simulink model "biomass"  (R2017a)
settings: Solver=VariableStepAuto  StartTime=0.0  StopTime=300  RelTol=1e-3
undefined symbols (not defined in the file): ba, bh, fp
settings Model: Creator=pum  LastModifiedBy=pum

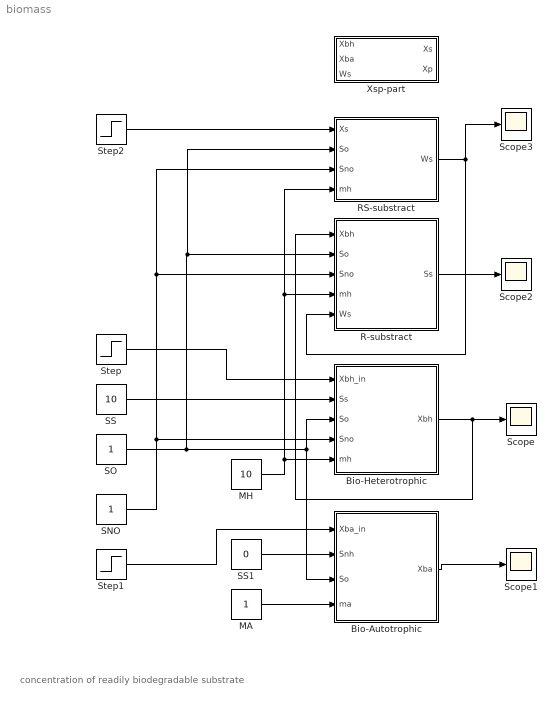
== system biomass ==
  note: concentration of readily biodegradable substrate
  Bio-Autotrophic : Subsystem  mask{Xba0=0, ba=1, Knh=3, Koa=5}
      mask prompts: Xba0 "Initialvalue"; ba "Ba cofficient"
  Bio-Heterotrophic : Subsystem  mask{Xbh0=0, bh=1, ng=1, Ks=0.1, Koh=0.1, Kno=0.3}
      mask prompts: Xbh0 "Initialvalue"; bh "Bh cofficient"; ng "Ng coefficient"
  MA : Constant
  MH : Constant  Value=10
  R-substract : Subsystem  mask{Y_h=50, ng=1, Ks=0.1, Koh=0.1, Kno=0.3}
  RS-substract : Subsystem  mask{kh=1, nh=1, Ks=0.1, Koh=0.1, Kno=0.3}
      mask prompts: nh "Ng"
  SNO : Constant
  SO : Constant
  SS : Constant  Value=10
  SS1 : Constant  Value=0
  Scope{,1..3} (4 alike) : Scope
  Step : Step  SampleTime=0
  Step1 : Step  SampleTime=0
  Step2 : Step  SampleTime=0
  Xsp-part : Subsystem
  wires:
  MH/1 -> RS-substract/4(mh), R-substract/4(mh), Bio-Heterotrophic/5(mh)
  SO/1 -> RS-substract/2(So), R-substract/2(So), Bio-Heterotrophic/3(So), Bio-Autotrophic/3(So)
  SNO/1 -> RS-substract/3(Sno), R-substract/3(Sno), Bio-Heterotrophic/4(Sno)
  Step/1 -> Bio-Heterotrophic/1(Xbh_in)
  MA/1 -> Bio-Autotrophic/4(ma)
  Step1/1 -> Bio-Autotrophic/1(Xba_in)
  Bio-Autotrophic/1(Xba) -> Scope1/1
  SS/1 -> Bio-Heterotrophic/2(Ss)
  SS1/1 -> Bio-Autotrophic/2(Snh)
  R-substract/1(Ss) -> Scope2/1
  Bio-Heterotrophic/1(Xbh) -> R-substract/1(Xbh), Scope/1
  RS-substract/1(Ws) -> Scope3/1, R-substract/5(Ws)
  Step2/1 -> RS-substract/1(Xs)

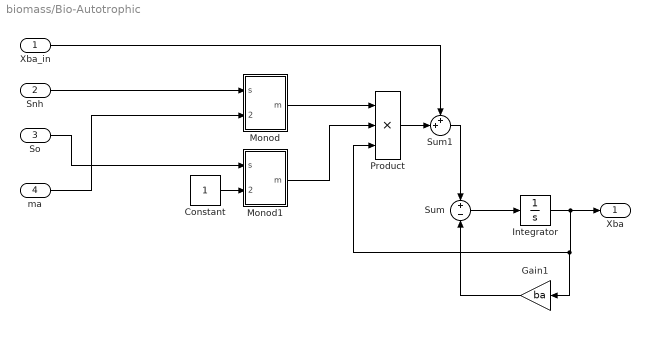
== system biomass/Bio-Autotrophic ==
  Xba_in : Inport
  Snh : Inport  Port=2
  So : Inport  Port=3
  ma : Inport  Port=4
  Constant : Constant
  Gain1 : Gain  Gain=ba
  Integrator : Integrator  InitialCondition=Xba0
  Monod : Subsystem  mask{K=Knh}
      mask prompts: K "Half-speed coeffcient"
  Monod1 : Subsystem  mask{K=Koa}
      mask prompts: K "Half-speed coeffcient"
  Product : Product  Inputs=3
  Sum : Sum  Inputs=+-
  Sum1 : Sum  Inputs=++|
  Xba : Outport
  wires:
  Integrator/1 -> Gain1/1, Product/3, Xba/1
  Snh/1 -> Monod/1(s)
  Monod1/1(m) -> Product/2
  Sum/1 -> Integrator/1
  Product/1 -> Sum1/2
  ma/1 -> Monod/2(m_max)
  Constant/1 -> Monod1/2(m_max)
  So/1 -> Monod1/1(s)
  Monod/1(m) -> Product/1
  Gain1/1 -> Sum/2
  Sum1/1 -> Sum/1
  Xba_in/1 -> Sum1/1

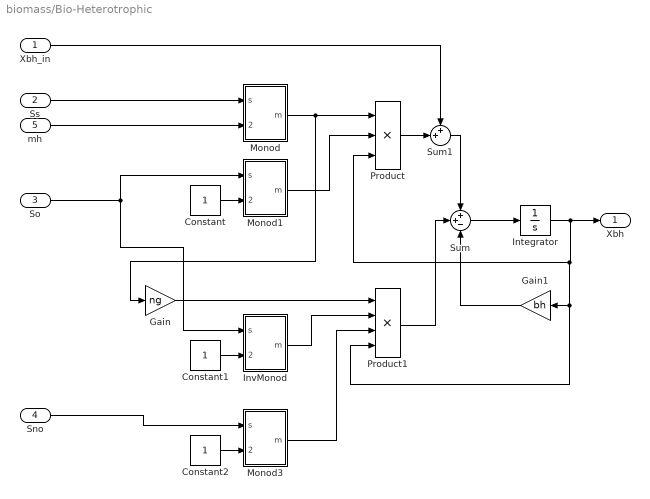
== system biomass/Bio-Heterotrophic ==
  Xbh_in : Inport
  Ss : Inport  Port=2
  So : Inport  Port=3
  Sno : Inport  Port=4
  mh : Inport  Port=5
  Constant : Constant
  Constant1 : Constant
  Constant2 : Constant
  Gain : Gain  Gain=ng
  Gain1 : Gain  Gain=bh
  Integrator : Integrator  InitialCondition=Xbh0
  InvMonod : Subsystem  mask{K=Koh}
      mask prompts: K "Half-speed coeffcient"
  Monod : Subsystem  mask{K=Ks}
      mask prompts: K "Half-speed coeffcient"
  Monod1 : Subsystem  mask{K=Koh}
      mask prompts: K "Half-speed coeffcient"
  Monod3 : Subsystem  mask{K=Kno}
      mask prompts: K "Half-speed coeffcient"
  Product : Product  Inputs=3
  Product1 : Product  Inputs=4
  Sum : Sum  Inputs=++-
  Sum1 : Sum  Inputs=++|
  Xbh : Outport
  wires:
  Integrator/1 -> Gain1/1, Product1/4, Product/3, Xbh/1
  Ss/1 -> Monod/1(s)
  Monod1/1(m) -> Product/2
  Sum/1 -> Integrator/1
  Product/1 -> Sum1/2
  mh/1 -> Monod/2(m_max)
  Constant/1 -> Monod1/2(m_max)
  So/1 -> InvMonod/1(s), Monod1/1(s)
  Monod/1(m) -> Gain/1, Product/1
  Sno/1 -> Monod3/1(s)
  Constant2/1 -> Monod3/2(m_max)
  Monod3/1(m) -> Product1/3
  Product1/1 -> Sum/2
  Gain/1 -> Product1/1
  Gain1/1 -> Sum/3
  Sum1/1 -> Sum/1
  Xbh_in/1 -> Sum1/1
  InvMonod/1(m) -> Product1/2
  Constant1/1 -> InvMonod/2(m_max)

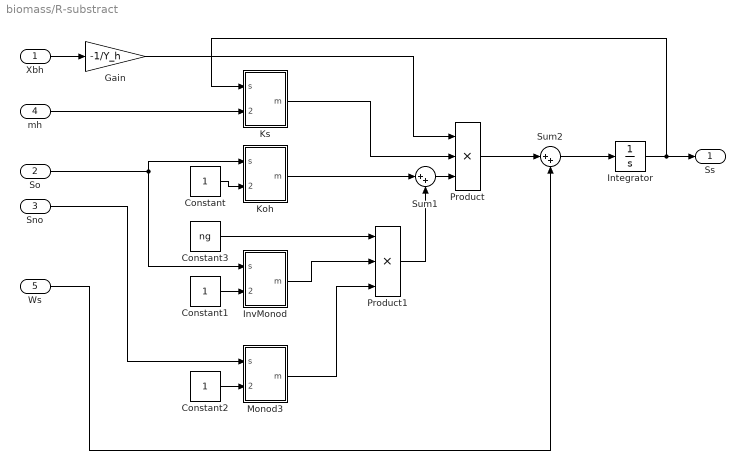
== system biomass/R-substract ==
  Xbh : Inport
  So : Inport  Port=2
  Sno : Inport  Port=3
  mh : Inport  Port=4
  Ws : Inport  Port=5
  Constant : Constant
  Constant1 : Constant
  Constant2 : Constant
  Constant3 : Constant  Value=ng
  Gain : Gain  Gain=-1/Y_h
  Integrator : Integrator
  InvMonod : Subsystem  mask{K=Koh}
      mask prompts: K "Half-speed coeffcient"
  Koh : Subsystem  mask{K=Koh}
      mask prompts: K "Half-speed coeffcient"
  Ks : Subsystem  mask{K=Ks}
      mask prompts: K "Half-speed coeffcient"
  Monod3 : Subsystem  mask{K=Kno}
      mask prompts: K "Half-speed coeffcient"
  Product : Product  Inputs=3
  Product1 : Product  Inputs=3
  Sum1 : Sum  Inputs=|++
  Sum2 : Sum  Inputs=|++
  Ss : Outport
  wires:
  Integrator/1 -> Ks/1(s), Ss/1
  Constant/1 -> Koh/2(m_max)
  Sno/1 -> Monod3/1(s)
  Constant2/1 -> Monod3/2(m_max)
  Monod3/1(m) -> Product1/3
  Constant3/1 -> Product1/1
  InvMonod/1(m) -> Product1/2
  Constant1/1 -> InvMonod/2(m_max)
  So/1 -> Koh/1(s), InvMonod/1(s)
  Product1/1 -> Sum1/2
  Koh/1(m) -> Sum1/1
  Sum1/1 -> Product/3
  Ks/1(m) -> Product/2
  Xbh/1 -> Gain/1
  Product/1 -> Sum2/1
  mh/1 -> Ks/2(m_max)
  Gain/1 -> Product/1
  Sum2/1 -> Integrator/1
  Ws/1 -> Sum2/2

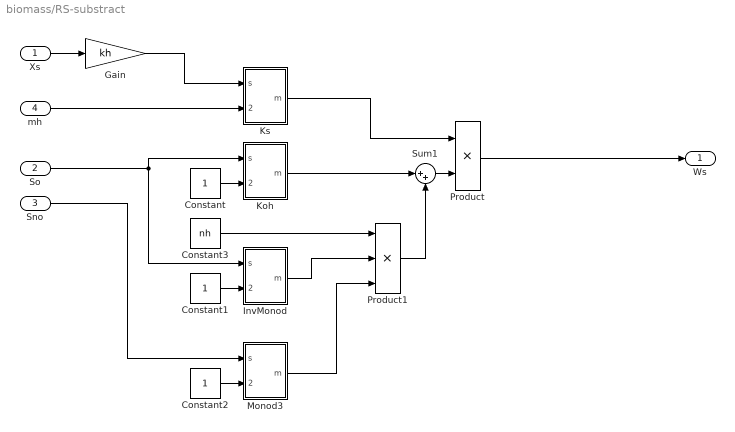
== system biomass/RS-substract ==
  Xs : Inport
  So : Inport  Port=2
  Sno : Inport  Port=3
  mh : Inport  Port=4
  Constant : Constant
  Constant1 : Constant
  Constant2 : Constant
  Constant3 : Constant  Value=nh
  Gain : Gain  Gain=kh
  InvMonod : Subsystem  mask{K=Koh}
      mask prompts: K "Half-speed coeffcient"
  Koh : Subsystem  mask{K=Koh}
      mask prompts: K "Half-speed coeffcient"
  Ks : Subsystem  mask{K=Ks}
      mask prompts: K "Half-speed coeffcient"
  Monod3 : Subsystem  mask{K=Kno}
      mask prompts: K "Half-speed coeffcient"
  Product : Product
  Product1 : Product  Inputs=3
  Sum1 : Sum  Inputs=|++
  Ws : Outport
  wires:
  Product/1 -> Ws/1
  Constant/1 -> Koh/2(m_max)
  Sno/1 -> Monod3/1(s)
  Constant2/1 -> Monod3/2(m_max)
  Monod3/1(m) -> Product1/3
  Constant3/1 -> Product1/1
  InvMonod/1(m) -> Product1/2
  Constant1/1 -> InvMonod/2(m_max)
  So/1 -> Koh/1(s), InvMonod/1(s)
  Product1/1 -> Sum1/2
  Koh/1(m) -> Sum1/1
  Sum1/1 -> Product/2
  Ks/1(m) -> Product/1
  Xs/1 -> Gain/1
  mh/1 -> Ks/2(m_max)
  Gain/1 -> Ks/1(s)

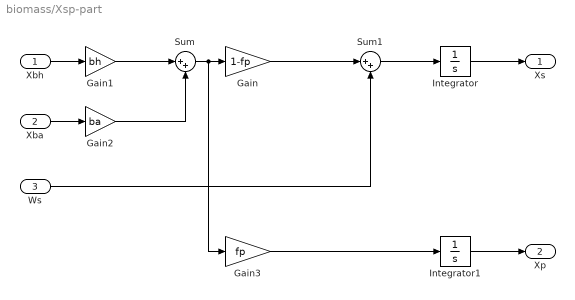
== system biomass/Xsp-part ==
  Xbh : Inport
  Xba : Inport  Port=2
  Ws : Inport  Port=3
  Gain : Gain  Gain=1-fp
  Gain1 : Gain  Gain=bh
  Gain2 : Gain  Gain=ba
  Gain3 : Gain  Gain=fp
  Integrator : Integrator
  Integrator1 : Integrator
  Sum : Sum  Inputs=|++
  Sum1 : Sum  Inputs=|++
  Xs : Outport
  Xp : Outport  Port=2
  wires:
  Xbh/1 -> Gain1/1
  Integrator/1 -> Xs/1
  Sum1/1 -> Integrator/1
  Xba/1 -> Gain2/1
  Gain2/1 -> Sum/2
  Gain1/1 -> Sum/1
  Gain/1 -> Sum1/1
  Ws/1 -> Sum1/2
  Sum/1 -> Gain3/1, Gain/1
  Integrator1/1 -> Xp/1
  Gain3/1 -> Integrator1/1

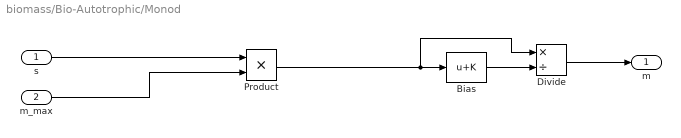
== system biomass/Bio-Autotrophic/Monod ==
  s : Inport
  m_max : Inport  Port=2
  Bias : Bias  Bias=K
  Divide : Product  Inputs=*/
  Product : Product
  m : Outport
  wires:
  Bias/1 -> Divide/2
  Divide/1 -> m/1
  Product/1 -> Divide/1, Bias/1
  s/1 -> Product/1
  m_max/1 -> Product/2

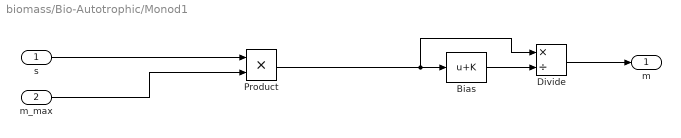
== system biomass/Bio-Autotrophic/Monod1 ==
  s : Inport
  m_max : Inport  Port=2
  Bias : Bias  Bias=K
  Divide : Product  Inputs=*/
  Product : Product
  m : Outport
  wires:
  Bias/1 -> Divide/2
  Divide/1 -> m/1
  Product/1 -> Divide/1, Bias/1
  s/1 -> Product/1
  m_max/1 -> Product/2

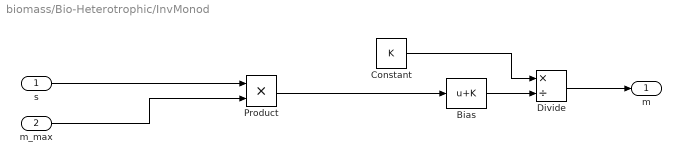
== system biomass/Bio-Heterotrophic/InvMonod ==
  s : Inport
  m_max : Inport  Port=2
  Bias : Bias  Bias=K
  Constant : Constant  Value=K
  Divide : Product  Inputs=*/
  Product : Product
  m : Outport
  wires:
  Bias/1 -> Divide/2
  Divide/1 -> m/1
  Product/1 -> Bias/1
  s/1 -> Product/1
  m_max/1 -> Product/2
  Constant/1 -> Divide/1

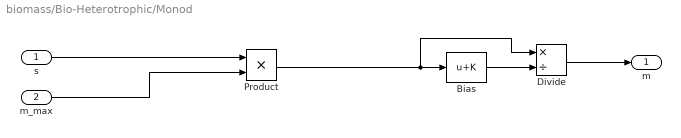
== system biomass/Bio-Heterotrophic/Monod ==
  s : Inport
  m_max : Inport  Port=2
  Bias : Bias  Bias=K
  Divide : Product  Inputs=*/
  Product : Product
  m : Outport
  wires:
  Bias/1 -> Divide/2
  Divide/1 -> m/1
  Product/1 -> Divide/1, Bias/1
  s/1 -> Product/1
  m_max/1 -> Product/2

== system biomass/Bio-Heterotrophic/Monod1 ==
  s : Inport
  m_max : Inport  Port=2
  Bias : Bias  Bias=K
  Divide : Product  Inputs=*/
  Product : Product
  m : Outport
  wires:
  Bias/1 -> Divide/2
  Divide/1 -> m/1
  Product/1 -> Divide/1, Bias/1
  s/1 -> Product/1
  m_max/1 -> Product/2

== system biomass/Bio-Heterotrophic/Monod3 ==
  s : Inport
  m_max : Inport  Port=2
  Bias : Bias  Bias=K
  Divide : Product  Inputs=*/
  Product : Product
  m : Outport
  wires:
  Bias/1 -> Divide/2
  Divide/1 -> m/1
  Product/1 -> Divide/1, Bias/1
  s/1 -> Product/1
  m_max/1 -> Product/2

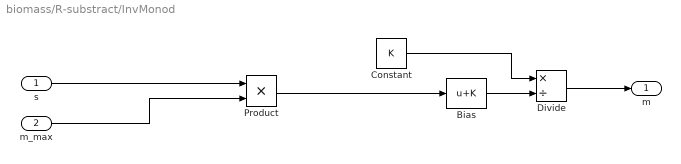
== system biomass/R-substract/InvMonod ==
  s : Inport
  m_max : Inport  Port=2
  Bias : Bias  Bias=K
  Constant : Constant  Value=K
  Divide : Product  Inputs=*/
  Product : Product
  m : Outport
  wires:
  Bias/1 -> Divide/2
  Divide/1 -> m/1
  Product/1 -> Bias/1
  s/1 -> Product/1
  m_max/1 -> Product/2
  Constant/1 -> Divide/1

== system biomass/R-substract/Koh ==
  s : Inport
  m_max : Inport  Port=2
  Bias : Bias  Bias=K
  Divide : Product  Inputs=*/
  Product : Product
  m : Outport
  wires:
  Bias/1 -> Divide/2
  Divide/1 -> m/1
  Product/1 -> Divide/1, Bias/1
  s/1 -> Product/1
  m_max/1 -> Product/2

== system biomass/R-substract/Ks ==
  s : Inport
  m_max : Inport  Port=2
  Bias : Bias  Bias=K
  Divide : Product  Inputs=*/
  Product : Product
  m : Outport
  wires:
  Bias/1 -> Divide/2
  Divide/1 -> m/1
  Product/1 -> Divide/1, Bias/1
  s/1 -> Product/1
  m_max/1 -> Product/2

== system biomass/R-substract/Monod3 ==
  s : Inport
  m_max : Inport  Port=2
  Bias : Bias  Bias=K
  Divide : Product  Inputs=*/
  Product : Product
  m : Outport
  wires:
  Bias/1 -> Divide/2
  Divide/1 -> m/1
  Product/1 -> Divide/1, Bias/1
  s/1 -> Product/1
  m_max/1 -> Product/2

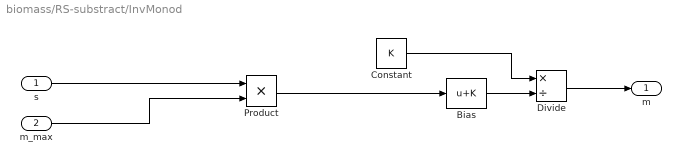
== system biomass/RS-substract/InvMonod ==
  s : Inport
  m_max : Inport  Port=2
  Bias : Bias  Bias=K
  Constant : Constant  Value=K
  Divide : Product  Inputs=*/
  Product : Product
  m : Outport
  wires:
  Bias/1 -> Divide/2
  Divide/1 -> m/1
  Product/1 -> Bias/1
  s/1 -> Product/1
  m_max/1 -> Product/2
  Constant/1 -> Divide/1

== system biomass/RS-substract/Koh ==
  s : Inport
  m_max : Inport  Port=2
  Bias : Bias  Bias=K
  Divide : Product  Inputs=*/
  Product : Product
  m : Outport
  wires:
  Bias/1 -> Divide/2
  Divide/1 -> m/1
  Product/1 -> Divide/1, Bias/1
  s/1 -> Product/1
  m_max/1 -> Product/2

== system biomass/RS-substract/Ks ==
  s : Inport
  m_max : Inport  Port=2
  Bias : Bias  Bias=K
  Divide : Product  Inputs=*/
  Product : Product
  m : Outport
  wires:
  Bias/1 -> Divide/2
  Divide/1 -> m/1
  Product/1 -> Divide/1, Bias/1
  s/1 -> Product/1
  m_max/1 -> Product/2

== system biomass/RS-substract/Monod3 ==
  s : Inport
  m_max : Inport  Port=2
  Bias : Bias  Bias=K
  Divide : Product  Inputs=*/
  Product : Product
  m : Outport
  wires:
  Bias/1 -> Divide/2
  Divide/1 -> m/1
  Product/1 -> Divide/1, Bias/1
  s/1 -> Product/1
  m_max/1 -> Product/2
